simulink model "Labo2_Parte1_simu"  (R2025b)
settings: Solver=FixedStepAuto  StartTime=0.0  StopTime=60  RelTol=1e-3
libraries: arduinolib x8, arduinosensorlib x1
settings Model: ExtModeTrigDuration=2  Creator=UCB  LastModifiedBy=UCB
settings SolverCC: AutoInsertRateTranBlk=on
settings OptimizationCC: EnhancedBackFolding=on  PassReuseOutputArgsAs=Individual arguments  ZeroExternalMemoryAtStartup=off  ZeroInternalMemoryAtStartup=off  MaxStackSize=64  OptimizeBlockOrder=speed  DifferentSizesBufferReuse=on  OptimizationCustomize=off  EfficientTunableParamExpr=on
settings DebuggingCC: ParameterTunabilityLossMsg=error
settings HardwareCC: ProdBitPerInt=16.0  ProdBitPerPointer=16.0  ProdBitPerSizeT=16.0  ProdBitPerPtrDiffT=16.0  ProdLargestAtomicFloat=None  ProdWordSize=8.0  ProdHWDeviceType=Atmel->AVR
settings SFSimCC: MATLABDynamicMemAlloc=off
settings RTWCC: SystemTargetFile=ert.tlc  HardwareBoard=Arduino Mega 2560  TemplateMakefile=ert_default_tmf  Toolchain=Arduino AVR  Description=Embedded Coder
settings CodeAppCC: ForceParamTrailComments=on  IgnoreCustomStorageClasses=off  OperatorAnnotations=on  SimulinkDataObjDesc=on  SFDataObjDesc=on  InsertBlockDesc=on
settings ERTTargetCC: ExtModeTransport=3.0  ExtModeStaticAlloc=on  ExtModeAutomaticAllocSize=off  ExtModeStaticAllocSize=2048.0  ExtModeMexFile=ext_xcp  ExtModeIntrfLevel=Level2 - Open  InlinedParameterPlacement=Hierarchical  DynamicArrayContainerType=coder::array  SupportContinuousTime=on  SupportVariableSizeSignals=on

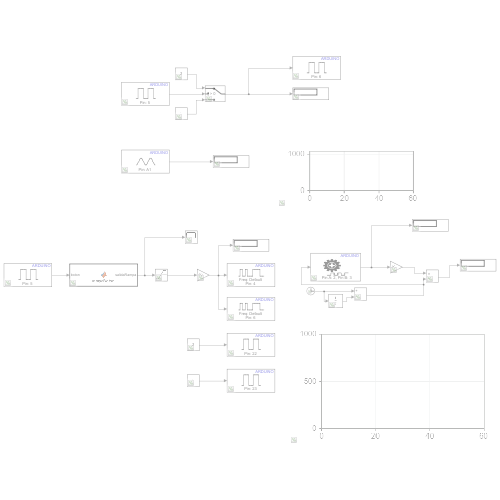
[thumbnail: Simulink's stored preview of the top-level diagram]
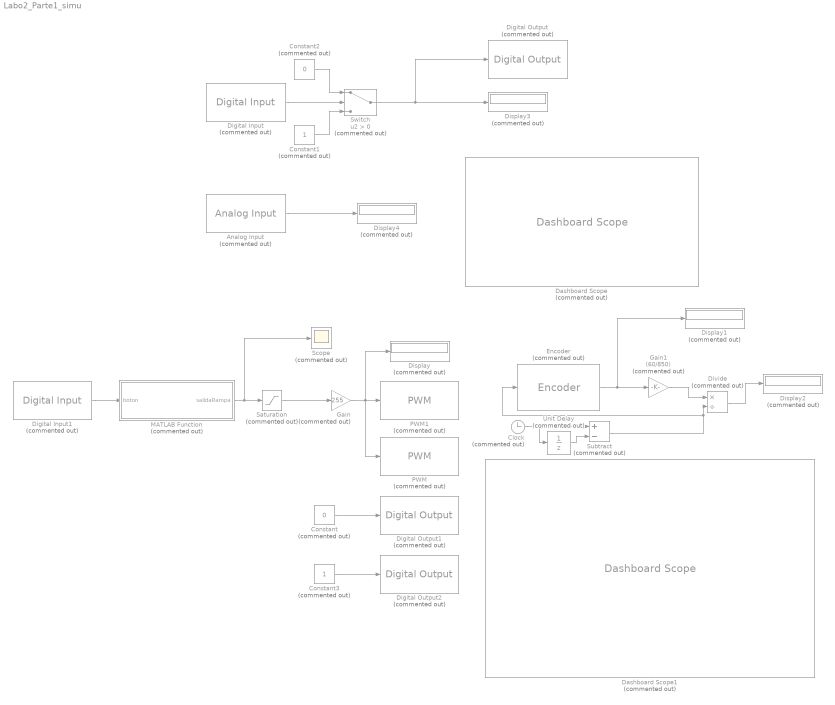
== system Labo2_Parte1_simu ==
  Analog Input : arduinolib/Analog Input  Commented=on  pinNumber=1  ReadResultsOnly=off  ConversionTriggerSource=Software  ExternalTriggerType=uint32( 0 )  OutputDataType=uint16  EnableConversionCompleteNotify=off  EnableOuputStatus=off  SampleTime=-1  blockPlatform=arduino
  Clock : Clock  Commented=on
  Constant : Constant  Commented=on  Value=0
  Constant1 : Constant  Commented=on  OutDataTypeStr=boolean
  Constant2 : Constant  Commented=on  Value=0  OutDataTypeStr=boolean
  Constant3 : Constant  Commented=on
  Dashboard Scope : DashboardScope  Commented=on  Ymin=0  Ymax=1100  FontColor=[0.0, 0.0, 0.0]
  Dashboard Scope1 : DashboardScope  Commented=on  Ymin=0  Ymax=1000  FontColor=[0.0, 0.0, 0.0]
  Digital Input : arduinolib/Digital Input  Commented=on  pinNumber=5  mode=Default  Direction=input  SampleTime=0.1  blockPlatform=arduino
  Digital Input1 : arduinolib/Digital Input  Commented=on  pinNumber=5  mode=Default  Direction=input  SampleTime=0.1  blockPlatform=arduino
  Digital Output : arduinolib/Digital Output  Commented=on  pinNumber=6  Direction=output  blockPlatform=arduino
  Digital Output1 : arduinolib/Digital Output  Commented=on  pinNumber=22  Direction=output  blockPlatform=arduino
  Digital Output2 : arduinolib/Digital Output  Commented=on  pinNumber=23  Direction=output  blockPlatform=arduino
  Display{,1..4} (5 alike) : Display  Commented=on
  Divide : Product  Commented=on  Inputs=*/
  Encoder : arduinosensorlib/Encoder  Commented=on  InputA=2  InputB=3  Mode=Reset by external signal  SampleTime=-1
  Gain : Gain  Commented=on  Gain=255
  Gain1 : Gain  Commented=on  Gain=(60/850)
  MATLAB Function : MATLAB Function  Commented=on  TreatAsAtomicUnit=on
  PWM : arduinolib/PWM  Commented=on  pinNumber=6  frequencyType=Default  desiredFrequency=490.2  achievableFrequency=490.2
  PWM1 : arduinolib/PWM  Commented=on  pinNumber=4  frequencyType=Default  desiredFrequency=490.2  achievableFrequency=490.2
  Saturation : Saturate  Commented=on  LowerLimit=0
  Scope : Scope  Commented=on
      settings: ActiveDisplayYMinimum=-1  ActiveDisplayYMaximum=1
  Subtract : Sum  Commented=on  Inputs=+-
  Switch : Switch  Commented=on  Criteria=u2 > Threshold  OutDataTypeStr=boolean  SaturateOnIntegerOverflow=off  InputSameDT=off
  Unit Delay : UnitDelay  Commented=on  SampleTime=-1  HasFrameUpgradeWarning=on
  wires:
  Encoder/1 -> Gain1/1, Display1/1
  Digital Input/1 -> Switch/2
  Switch/1 -> Digital Output/1, Display3/1
  Constant1/1 -> Switch/3
  Constant2/1 -> Switch/1
  Analog Input/1 -> Display4/1
  MATLAB Function/1(salidaRampa) -> Saturation/1, Scope/1
  Digital Input1/1 -> MATLAB Function/1(boton)
  Gain/1 -> Display/1, PWM/1, PWM1/1
  Saturation/1 -> Gain/1
  Constant/1 -> Digital Output1/1
  Constant3/1 -> Digital Output2/1
  Divide/1 -> Display2/1
  Clock/1 -> Subtract/1, Unit Delay/1
  Unit Delay/1 -> Subtract/2
  Subtract/1 -> Divide/2, Encoder/1
  Gain1/1 -> Divide/1

== matlab function Labo2_Parte1_simu/MATLAB Function ==
  data: boton input; salidaRampa output
function salidaRampa = rampaBoton(boton)
% Entradas:
%   boton       : Booleano (true/1 = presionado, false/0 = suelto)
% Salida:
%   salidaRampa : Rampa entre 0.0 y 1.0 sin retraso al soltar o presionar

    persistent valorRampa
    if isempty(valorRampa)
        valorRampa = 0.0;
    end

    dt = 0.01;            % Sample time del solver de Simulink
    tiempoTransicion = 5; % Segundos para ir de 0 a 1
    paso = dt / tiempoTransicion;

    % 1. Calcular el valor potencial
    if boton
        nuevoValor = valorRampa + paso;
    else
        nuevoValor = valorRampa - paso;
    end

    % 2. RECORTAR Y REASIGNAR A LA VARIABLE PERSISTENTE
    % Esto fuerza a que 'valorRampa' NUNCA supere 1.0 ni sea menor a 0.0
    if nuevoValor > 0.5
        valorRampa = 0.5;
    elseif nuevoValor < 0.0
        valorRampa = 0.0;
    else
        valorRampa = nuevoValor;
    end

    % 3. Salida
    salidaRampa = valorRampa;
end
